simulink model "rotation_integration_rpyD_test"  (Simulink 8.5)
settings: Solver=ode4  StartTime=0.0  StopTime=10.0  FixedStep=1e-3  RelTol=Tolerance
values from neighbouring files (symbols this model uses):
  A = [0 1 -0.5]    [rotation_integration_comparison.m]
libraries: rigid_body_kinematics x1, rotation_test_input_library x1
settings Model: Creator=schappler  LastModifiedBy=Vorndamme
settings DataIOCC: LimitDataPoints=off  SaveFormat=StructureWithTime  SignalLoggingSaveFormat=Dataset  SignalLogging=off
settings OptimizationCC: ExpressionDepthLimit=128
settings DebuggingCC: UnderspecifiedInitializationDetection=Simplified  MergeDetectMultiDrivingBlocksExec=error  FcnCallInpInsideContextMsg=EnableAllAsError  StateNameClashWarn=none
settings GRTTargetCC: CombineOutputUpdateFcns=on  GRTInterface=off

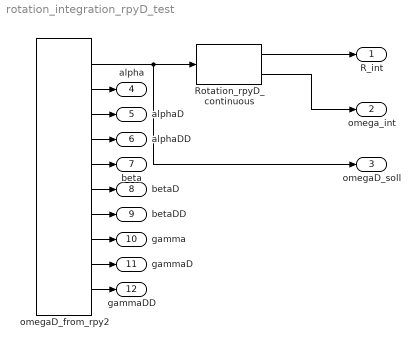
== system rotation_integration_rpyD_test ==
  Rotation_rpyD_continuous : rigid_body_kinematics/Rotation_rpyD_continuous  R_0E_t0=R_t0  omega0_t0=omega0_t0
  omegaD_from_rpy2 : rotation_test_input_library/omegaD_from_rpy  A=A  f=f  rpy_offsetts=rpy_offsets  rpy_phases=rpy_phases
  R_int : Outport
  omega_int : Outport  Port=2
  omegaD_soll : Outport  Port=3
  alpha : Outport  Port=4
  alphaD : Outport  Port=5
  alphaDD : Outport  Port=6
  beta : Outport  Port=7
  betaD : Outport  Port=8
  betaDD : Outport  Port=9
  gamma : Outport  Port=10
  gammaD : Outport  Port=11
  gammaDD : Outport  Port=12
  wires:
  omegaD_from_rpy2/1 -> Rotation_rpyD_continuous/1, omegaD_soll/1
  Rotation_rpyD_continuous/1 -> R_int/1
  Rotation_rpyD_continuous/2 -> omega_int/1
  omegaD_from_rpy2/2 -> alpha/1
  omegaD_from_rpy2/3 -> alphaD/1
  omegaD_from_rpy2/4 -> alphaDD/1
  omegaD_from_rpy2/5 -> beta/1
  omegaD_from_rpy2/6 -> betaD/1
  omegaD_from_rpy2/7 -> betaDD/1
  omegaD_from_rpy2/8 -> gamma/1
  omegaD_from_rpy2/9 -> gammaD/1
  omegaD_from_rpy2/10 -> gammaDD/1
